simulink library "StdAnimationLibrary_R2020b"  (R2020b)
settings: Solver=VariableStepAuto  StartTime=0.0  StopTime=10.0  RelTol=1e-3
libraries: simulink x8
settings Model: Creator=mchawa  LastModifiedBy=oashraf
settings DataIOCC: ReturnWorkspaceOutputs=off
settings DebuggingCC: ArithmeticOperatorsInVariantConditions=warning
settings SFSimCC: SimUseLocalCustomCode=off  CustomCodeUndefinedFunction=UseInterfaceOnly
settings RTWCC: RTWUseLocalCustomCode=off

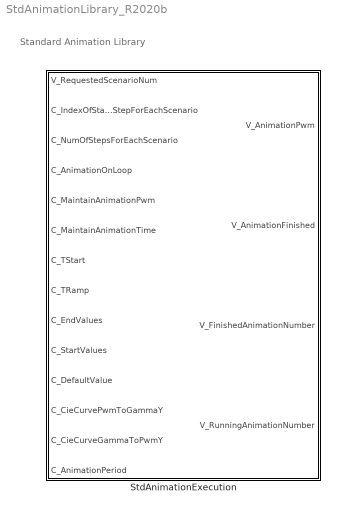
== system StdAnimationLibrary_R2020b ==
  note: Standard Animation Library
  StdAnimationExecution : Subsystem  Description=|
      | S___122_135
      | S___122_242
      | S___122_240

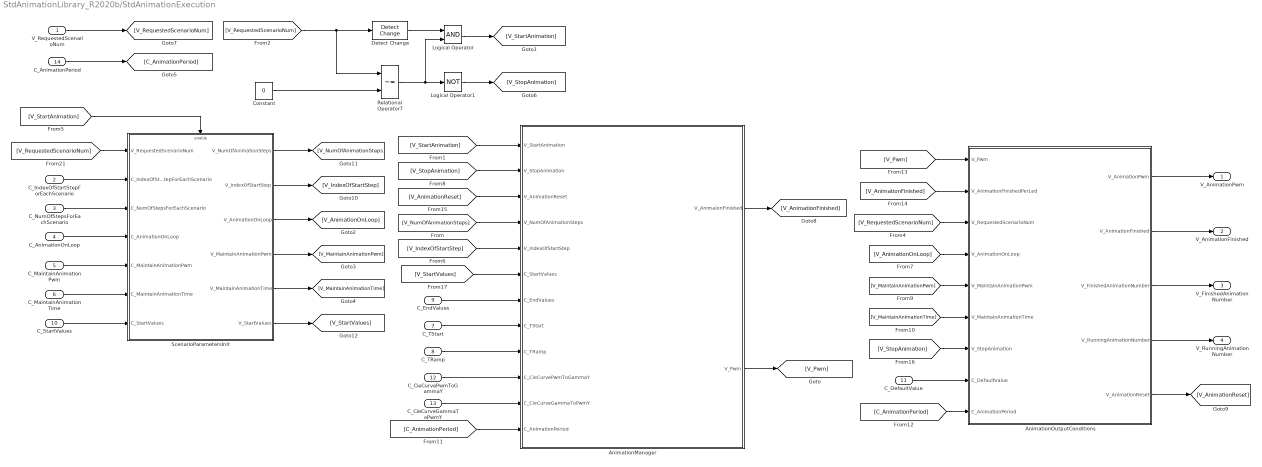
== system StdAnimationLibrary_R2020b/StdAnimationExecution ==
  V_RequestedScenarioNum : Inport
  C_IndexOfStartStepForEachScenario : Inport  Port=2
  C_NumOfStepsForEachScenario : Inport  Port=3
  C_AnimationOnLoop : Inport  Port=4
  C_MaintainAnimationPwm : Inport  Port=5
  C_MaintainAnimationTime : Inport  Port=6
  C_TStart : Inport  Port=7
  C_TRamp : Inport  Port=8
  C_EndValues : Inport  Port=9
  C_StartValues : Inport  Port=10
  C_DefaultValue : Inport  Port=11
  C_CieCurvePwmToGammaY : Inport  Port=12
  C_CieCurveGammaToPwmY : Inport  Port=13
  C_AnimationPeriod : Inport  Port=14
  AnimationManager : Subsystem  TreatAsAtomicUnit=on
  AnimationOutputConditions : Subsystem  Description=|
      | S___122_237
      | S___122_244
  Constant : Constant  Value=0  OutDataTypeStr=uint8
  Detect Change : simulink/Logic and Bit Operations/Detect Change  vinit=0  OutDataTypeStr=boolean
  Logical Operator : Logic  AllPortsSameDT=off  OutDataTypeStr=boolean
  Logical Operator1 : Logic  Operator=NOT  AllPortsSameDT=off  OutDataTypeStr=boolean
  Relational Operator7 : RelationalOperator  Operator=~=  OutDataTypeStr=boolean  RndMeth=Simplest
  ScenarioParametersInit : Subsystem  TreatAsAtomicUnit=on
  V_AnimationPwm : Outport  VectorParamsAs1DForOutWhenUnconnected=off
  V_AnimationFinished : Outport  Port=2  VectorParamsAs1DForOutWhenUnconnected=off
  V_FinishedAnimationNumber : Outport  Port=3  VectorParamsAs1DForOutWhenUnconnected=off
  V_RunningAnimationNumber : Outport  Port=4  VectorParamsAs1DForOutWhenUnconnected=off
  wires:
  V_RequestedScenarioNum/1 -> [V_RequestedScenarioNum]
  [V_StartAnimation] -> AnimationManager/1(V_StartAnimation)
  C_EndValues/1 -> AnimationManager/7(C_EndValues)
  C_TStart/1 -> AnimationManager/8(C_TStart)
  [V_StopAnimation] -> AnimationManager/2(V_StopAnimation)
  C_TRamp/1 -> AnimationManager/9(C_TRamp)
  Constant/1 -> Relational Operator7/2
  C_CieCurveGammaToPwmY/1 -> AnimationManager/11(C_CieCurveGammaToPwmY)
  [V_RequestedScenarioNum] -> AnimationOutputConditions/3(V_RequestedScenarioNum)
  [V_RequestedScenarioNum] -> Relational Operator7/1, Detect Change/1
  C_IndexOfStartStepForEachScenario/1 -> ScenarioParametersInit/2(C_IndexOfStartStepForEachScenario)
  C_NumOfStepsForEachScenario/1 -> ScenarioParametersInit/3(C_NumOfStepsForEachScenario)
  C_DefaultValue/1 -> AnimationOutputConditions/8(C_DefaultValue)
  C_CieCurvePwmToGammaY/1 -> AnimationManager/10(C_CieCurvePwmToGammaY)
  [V_RequestedScenarioNum] -> ScenarioParametersInit/1(V_RequestedScenarioNum)
  ScenarioParametersInit/2(V_IndexOfStartStep) -> [V_IndexOfStartStep]
  ScenarioParametersInit/1(V_NumOfAnimationSteps) -> [V_NumOfAnimationSteps]
  [V_StartAnimation] -> ScenarioParametersInit/Enable
  [V_NumOfAnimationSteps] -> AnimationManager/4(V_NumOfAnimationSteps)
  [V_IndexOfStartStep] -> AnimationManager/5(V_IndexOfStartStep)
  C_AnimationOnLoop/1 -> ScenarioParametersInit/4(C_AnimationOnLoop)
  C_MaintainAnimationPwm/1 -> ScenarioParametersInit/5(C_MaintainAnimationPwm)
  C_MaintainAnimationTime/1 -> ScenarioParametersInit/6(C_MaintainAnimationTime)
  Detect Change/1 -> Logical Operator/1
  Relational Operator7/1 -> Logical Operator1/1, Logical Operator/2
  Logical Operator/1 -> [V_StartAnimation]
  Logical Operator1/1 -> [V_StopAnimation]
  ScenarioParametersInit/3(V_AnimationOnLoop) -> [V_AnimationOnLoop]
  ScenarioParametersInit/4(V_MaintainAnimationPwm) -> [V_MaintainAnimationPwm]
  ScenarioParametersInit/5(V_MaintainAnimationTime) -> [V_MaintainAnimationTime]
  [V_AnimationOnLoop] -> AnimationOutputConditions/4(V_AnimationOnLoop)
  [V_MaintainAnimationPwm] -> AnimationOutputConditions/5(V_MaintainAnimationPwm)
  [V_MaintainAnimationTime] -> AnimationOutputConditions/6(V_MaintainAnimationTime)
  C_AnimationPeriod/1 -> [C_AnimationPeriod]
  [C_AnimationPeriod] -> AnimationManager/12(C_AnimationPeriod)
  [C_AnimationPeriod] -> AnimationOutputConditions/9(C_AnimationPeriod)
  AnimationManager/2(V_Pwm) -> [V_Pwm]
  AnimationManager/1(V_AnimaionFinished) -> [V_AnimationFinished]
  [V_Pwm] -> AnimationOutputConditions/1(V_Pwm)
  [V_AnimationFinished] -> AnimationOutputConditions/2(V_AnimationFinishedPerLed)
  [V_AnimationReset] -> AnimationManager/3(V_AnimationReset)
  [V_StopAnimation] -> AnimationOutputConditions/7(V_StopAnimation)
  C_StartValues/1 -> ScenarioParametersInit/7(C_StartValues)
  ScenarioParametersInit/6(V_StartValues) -> [V_StartValues]
  [V_StartValues] -> AnimationManager/6(C_StartValues)
  AnimationOutputConditions/1(V_AnimationPwm) -> V_AnimationPwm/1
  AnimationOutputConditions/3(V_FinishedAnimationNumber) -> V_FinishedAnimationNumber/1
  AnimationOutputConditions/4(V_RunningAnimationNumber) -> V_RunningAnimationNumber/1
  AnimationOutputConditions/5(V_AnimationReset) -> [V_AnimationReset]
  AnimationOutputConditions/2(V_AnimationFinished) -> V_AnimationFinished/1

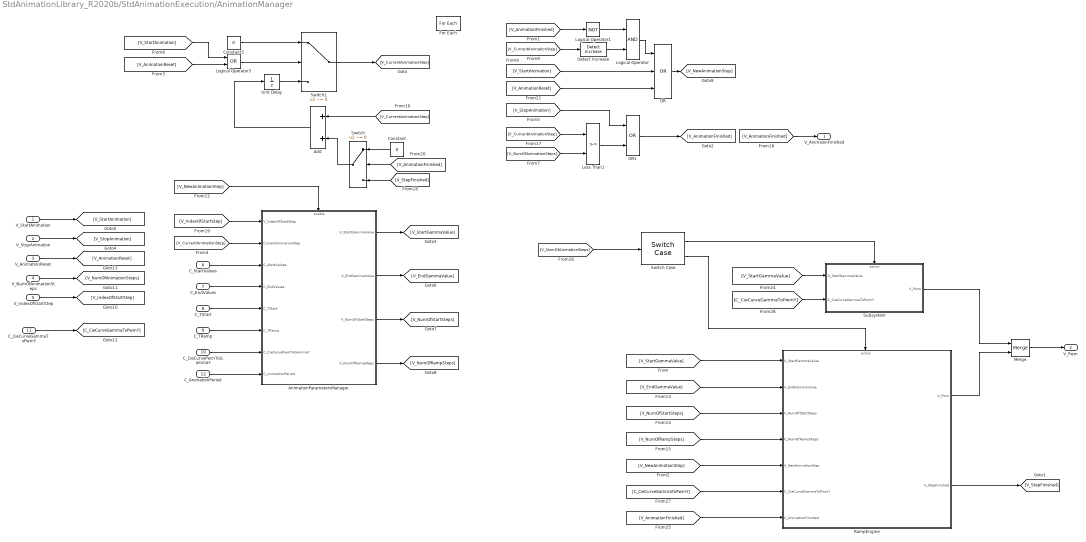
== system StdAnimationLibrary_R2020b/StdAnimationExecution/AnimationManager ==
  V_StartAnimation : Inport  OutDataTypeStr=boolean
  V_StopAnimation : Inport  Port=2  OutDataTypeStr=boolean
  V_AnimationReset : Inport  Port=3
  V_NumOfAnimationSteps : Inport  Port=4  Partition=on  PartitionDimension=2  PartitionWidth=1  PartitionOffset=0
  V_IndexOfStartStep : Inport  Port=5  Partition=on  PartitionDimension=2  PartitionWidth=1  PartitionOffset=0
  C_StartValues : Inport  Port=6  Partition=on  PartitionDimension=2  PartitionWidth=1  PartitionOffset=0
  C_EndValues : Inport  Port=7
  C_TStart : Inport  Port=8
  C_TRamp : Inport  Port=9
  C_CieCurvePwmToGammaY : Inport  Port=10
  C_CieCurveGammaToPwmY : Inport  Port=11
  C_AnimationPeriod : Inport  Port=12
  Add : Sum
  AnimationParametersManager : Subsystem  TreatAsAtomicUnit=on
  Constant : Constant  Value=0  OutDataTypeStr=uint8
  Constant5 : Constant  Value=0  OutDataTypeStr=uint8
  Detect Increase : simulink/Logic and Bit Operations/Detect Increase  vinit=0.0  OutDataTypeStr=boolean
  For Each : ForEach  DisableCoverage=on
  Less Than1 : RelationalOperator  OutDataTypeStr=boolean  RndMeth=Simplest
  Logical Operator : Logic  AllPortsSameDT=off  OutDataTypeStr=boolean
  Logical Operator1 : Logic  Operator=NOT  AllPortsSameDT=off  OutDataTypeStr=boolean
  Logical Operator3 : Logic  Operator=OR  AllPortsSameDT=off  OutDataTypeStr=boolean
  Merge : Merge
  OR : Logic  Operator=OR  Inputs=3  AllPortsSameDT=off  OutDataTypeStr=boolean
  OR1 : Logic  Operator=OR  AllPortsSameDT=off  OutDataTypeStr=boolean
  RampEngine : Subsystem
  Subsystem : Subsystem
  Switch : Switch  Criteria=u2 ~= 0
  Switch Case : SwitchCase  CaseConditions={0}
  Switch1 : Switch  Criteria=u2 ~= 0  OutDataTypeStr=Inherit: Inherit via back propagation  SaturateOnIntegerOverflow=on
  Unit Delay : UnitDelay  SampleTime=-1  HasFrameUpgradeWarning=on
  V_AnimaionFinished : Outport  ConcatenationDimension=1  VectorParamsAs1DForOutWhenUnconnected=off
  V_Pwm : Outport  Port=2  ConcatenationDimension=1  VectorParamsAs1DForOutWhenUnconnected=off
  wires:
  [V_CurrentAnimationStep] -> AnimationParametersManager/2(CurrentAnimationStep)
  Constant5/1 -> Switch1/1
  C_EndValues/1 -> AnimationParametersManager/4(C_EndValues)
  [V_StopAnimation] -> OR1/1
  C_TStart/1 -> AnimationParametersManager/5(C_TStart)
  C_TRamp/1 -> AnimationParametersManager/6(C_TRamp)
  V_StartAnimation/1 -> [V_StartAnimation]
  V_StopAnimation/1 -> [V_StopAnimation]
  C_StartValues/1 -> AnimationParametersManager/3(C_StartValues)
  Switch1/1 -> [V_CurrentAnimationStep]
  RampEngine/1(V_Pwm) -> Merge/2
  Add/1 -> Unit Delay/1
  [V_StartAnimation] -> OR/2
  [V_NewAnimationStep] -> AnimationParametersManager/Enable
  C_AnimationPeriod/1 -> AnimationParametersManager/8(C_AnimationPeriod)
  AnimationParametersManager/1(V_StartGammaValue) -> [V_StartGammaValue]
  AnimationParametersManager/2(V_EndGammaValue) -> [V_EndGammaValue]
  AnimationParametersManager/3(V_NumOfStartSteps) -> [V_NumOfStartSteps]
  AnimationParametersManager/4(V_NumOfRampSteps) -> [V_NumOfRampSteps]
  [V_NewAnimationStep] -> RampEngine/5(V_NewAnimationStep)
  [V_StartGammaValue] -> RampEngine/1(V_StartGammaValue)
  [V_EndGammaValue] -> RampEngine/2(V_EndGammaValue)
  [V_NumOfStartSteps] -> RampEngine/3(V_NumOfStartSteps)
  [V_NumOfRampSteps] -> RampEngine/4(V_NumOfRampSteps)
  [V_AnimationFinished] -> V_AnimaionFinished/1
  [V_CurrentAnimationStep] -> Detect Increase/1
  Logical Operator/1 -> OR/1
  Logical Operator1/1 -> Logical Operator/1
  [V_AnimationFinished] -> Logical Operator1/1
  RampEngine/2(V_StepFinished) -> [V_StepFinished]
  [V_CurrentAnimationStep] -> Add/1
  Unit Delay/1 -> Switch1/3
  Less Than1/1 -> OR1/2
  OR/1 -> [V_NewAnimationStep]
  OR1/1 -> [V_AnimationFinished]
  Detect Increase/1 -> Logical Operator/2
  [V_IndexOfStartStep] -> AnimationParametersManager/1(V_IndexOfStartStep)
  Switch/1 -> Add/2
  [V_StepFinished] -> Switch/3
  [V_AnimationFinished] -> Switch/2
  Constant/1 -> Switch/1
  [V_NumOfAnimationSteps] -> Less Than1/2
  [V_CurrentAnimationStep] -> Less Than1/1
  C_CieCurvePwmToGammaY/1 -> AnimationParametersManager/7(C_CieCurvePwmToGammaY)
  V_IndexOfStartStep/1 -> [V_IndexOfStartStep]
  V_NumOfAnimationSteps/1 -> [V_NumOfAnimationSteps]
  V_AnimationReset/1 -> [V_AnimationReset]
  Logical Operator3/1 -> Switch1/2
  [V_AnimationReset] -> Logical Operator3/2
  [V_StartAnimation] -> Logical Operator3/1
  [V_AnimationReset] -> OR/3
  Subsystem/1(V_Pwm) -> Merge/1
  [V_StartGammaValue] -> Subsystem/1(V_StartGammaValue)
  [V_NumOfAnimationSteps] -> Switch Case/1
  Switch Case/1 -> Subsystem/Action
  [V_AnimationFinished] -> RampEngine/7(V_AnimationFinished)
  Merge/1 -> V_Pwm/1
  C_CieCurveGammaToPwmY/1 -> [C_CieCurveGammaToPwmY]
  [C_CieCurveGammaToPwmY] -> RampEngine/6(C_CieCurveGammaToPwmY)
  [C_CieCurveGammaToPwmY] -> Subsystem/2(C_CieCurveGammaToPwmY)
  Switch Case/2 -> RampEngine/Action

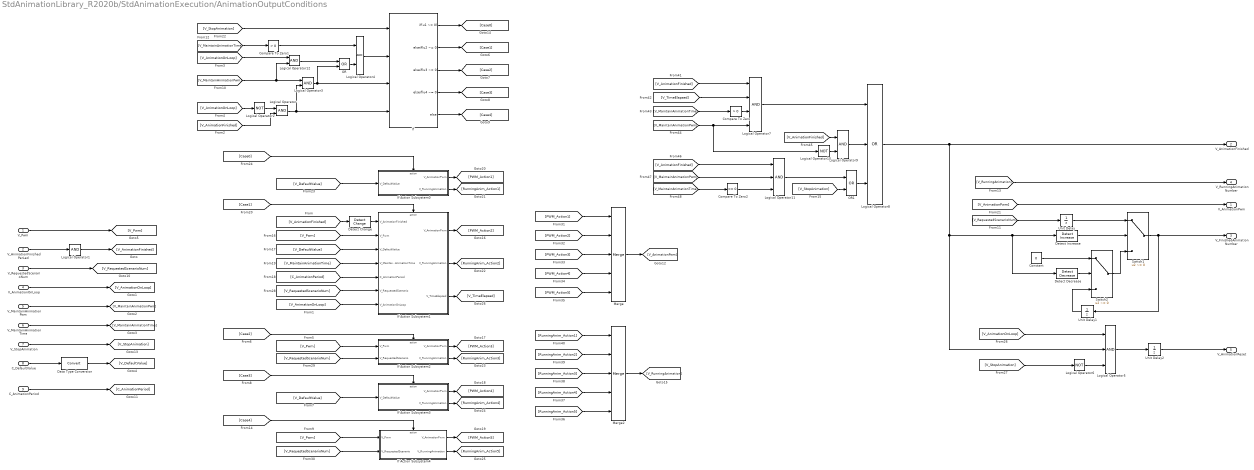
== system StdAnimationLibrary_R2020b/StdAnimationExecution/AnimationOutputConditions ==
  V_Pwm : Inport
  V_AnimationFinishedPerLed : Inport  Port=2
  V_RequestedScenarioNum : Inport  Port=3
  V_AnimationOnLoop : Inport  Port=4
  V_MaintainAnimationPwm : Inport  Port=5
  V_MaintainAnimationTime : Inport  Port=6
  V_StopAnimation : Inport  Port=7
  C_DefaultValue : Inport  Port=8
  C_AnimationPeriod : Inport  Port=9
  Compare To Zero : simulink/Logic and Bit Operations/Compare To Zero  relop=>  OutDataTypeStr=boolean
  Compare To Zero1 : simulink/Logic and Bit Operations/Compare To Zero  relop=>  OutDataTypeStr=boolean
  Compare To Zero2 : simulink/Logic and Bit Operations/Compare To Zero  relop===  OutDataTypeStr=boolean
  Constant : Constant  Value=0  OutDataTypeStr=uint8
  Data Type Conversion : DataTypeConversion
  Detect Change : simulink/Logic and Bit Operations/Detect Change  vinit=0  OutDataTypeStr=boolean
  Detect Decrease : simulink/Logic and Bit Operations/Detect Decrease  vinit=0.0  OutDataTypeStr=boolean
  Detect Increase : simulink/Logic and Bit Operations/Detect Increase  vinit=0.0  OutDataTypeStr=boolean
  If : If  NumInputs=4  IfExpression=u1 ~= 0  ElseIfExpressions=u2 ~= 0, u3 ~= 0, u4 ~= 0
  If Action Subsystem0 : Subsystem  TreatAsAtomicUnit=on
  If Action Subsystem1 : Subsystem  Description=S___122_238  TreatAsAtomicUnit=on
  If Action Subsystem2 : Subsystem  TreatAsAtomicUnit=on
  If Action Subsystem3 : Subsystem  TreatAsAtomicUnit=on
  If Action Subsystem4 : Subsystem  TreatAsAtomicUnit=on
  Logical Operator{,3..4,9,12} (5 alike) : Logic  AllPortsSameDT=off  OutDataTypeStr=boolean
  Logical Operator1 : Logic  Inputs=1  AllPortsSameDT=off  OutDataTypeStr=boolean
  Logical Operator10 : Logic  Operator=NOT  AllPortsSameDT=off  OutDataTypeStr=boolean
  Logical Operator11 : Logic  Inputs=3  AllPortsSameDT=off  OutDataTypeStr=boolean
  Logical Operator2 : Logic  Operator=NOT  AllPortsSameDT=off  OutDataTypeStr=boolean
  Logical Operator5 : Logic  Inputs=3  AllPortsSameDT=off  OutDataTypeStr=boolean
  Logical Operator6 : Logic  Operator=NOT  AllPortsSameDT=off  OutDataTypeStr=boolean
  Logical Operator7 : Logic  Inputs=4  AllPortsSameDT=off  OutDataTypeStr=boolean
  Logical Operator8 : Logic  Operator=OR  Inputs=3  AllPortsSameDT=off  OutDataTypeStr=boolean
  Merge : Merge  Inputs=5
  Merge2 : Merge  Inputs=5
  OR : Logic  Operator=OR  AllPortsSameDT=off  OutDataTypeStr=boolean
  OR1 : Logic  Operator=OR  AllPortsSameDT=off  OutDataTypeStr=boolean
  Switch1 : Switch  Criteria=u2 ~= 0
  Switch2 : Switch  Criteria=u2 ~= 0
  Unit Delay : UnitDelay  SampleTime=-1  HasFrameUpgradeWarning=on
  Unit Delay1 : UnitDelay  SampleTime=-1  HasFrameUpgradeWarning=on
  Unit Delay2 : UnitDelay  SampleTime=-1  HasFrameUpgradeWarning=on
  V_AnimationPwm : Outport
  V_AnimationFinished : Outport  Port=2
  V_FinishedAnimationNumber : Outport  Port=3
  V_RunningAnimationNumber : Outport  Port=4
  V_AnimationReset : Outport  Port=5
  wires:
  [V_StopAnimation] -> OR1/2
  Logical Operator11/1 -> OR1/1
  OR1/1 -> Logical Operator8/3
  V_AnimationFinishedPerLed/1 -> Logical Operator1/1
  V_RequestedScenarioNum/1 -> [V_RequestedScenarioNum]
  [V_RequestedScenarioNum] -> Unit Delay/1
  C_DefaultValue/1 -> Data Type Conversion/1
  Logical Operator1/1 -> [V_AnimationFinished]
  Unit Delay/1 -> Switch1/1
  Switch2/1 -> Switch1/3
  Switch1/1 -> V_FinishedAnimationNumber/1, Unit Delay1/1
  Unit Delay1/1 -> Switch2/3
  Detect Increase/1 -> Switch1/2
  Detect Decrease/1 -> Switch2/2
  Constant/1 -> Switch2/1
  [V_AnimationFinished] -> Logical Operator/2
  [V_AnimationOnLoop] -> Logical Operator2/1
  V_AnimationOnLoop/1 -> [V_AnimationOnLoop]
  V_MaintainAnimationPwm/1 -> [V_MaintainAnimationPwm]
  V_MaintainAnimationTime/1 -> [V_MaintainAnimationTime]
  Data Type Conversion/1 -> [V_DefaultValue]
  V_Pwm/1 -> [V_Pwm]
  Logical Operator2/1 -> Logical Operator/1
  [V_MaintainAnimationPwm] -> Logical Operator12/2, Logical Operator3/1
  Logical Operator3/1 -> OR/2, If/3
  [V_MaintainAnimationTime] -> Compare To Zero1/1
  Compare To Zero1/1 -> Logical Operator4/1
  If/5 -> [Case4]
  [V_Pwm] -> If Action Subsystem2/1(V_Pwm)
  [Case2] -> If Action Subsystem2/Action
  [V_DefaultValue] -> If Action Subsystem3/1(V_DefaultValue)
  [Case3] -> If Action Subsystem3/Action
  [V_Pwm] -> If Action Subsystem4/1(V_Pwm)
  [Case4] -> If Action Subsystem4/Action
  C_AnimationPeriod/1 -> [C_AnimationPeriod]
  [V_Pwm] -> If Action Subsystem1/2(V_Pwm)
  [V_DefaultValue] -> If Action Subsystem1/3(V_DefaultValue)
  [V_MaintainAnimationTime] -> If Action Subsystem1/4(V_MaintainAnimationTime)
  [C_AnimationPeriod] -> If Action Subsystem1/5(C_AnimationPeriod)
  [Case1] -> If Action Subsystem1/Action
  Merge/1 -> [V_AnimationPwm]
  [V_AnimationPwm] -> V_AnimationPwm/1
  V_StopAnimation/1 -> [V_StopAnimation]
  If/4 -> [Case3]
  If/1 -> [Case0]
  If/2 -> [Case1]
  If/3 -> [Case2]
  [V_StopAnimation] -> If/1
  Logical Operator4/1 -> If/2
  Logical Operator/1 -> Logical Operator3/2, If/4
  [V_DefaultValue] -> If Action Subsystem0/1(V_DefaultValue)
  [Case0] -> If Action Subsystem0/Action
  [V_AnimationOnLoop] -> Logical Operator5/1
  [V_StopAnimation] -> Logical Operator6/1
  Logical Operator6/1 -> Logical Operator5/3
  Logical Operator5/1 -> Unit Delay2/1
  Unit Delay2/1 -> V_AnimationReset/1
  [V_RunningAnimation] -> V_RunningAnimationNumber/1
  [V_RequestedScenarioNum] -> If Action Subsystem1/6(V_RequestedScenario)
  [V_RequestedScenarioNum] -> If Action Subsystem2/2(V_RequestedScenario)
  [V_RequestedScenarioNum] -> If Action Subsystem4/2(V_RequestedScenario)
  Merge2/1 -> [V_RunningAnimation]
  If Action Subsystem2/1(V_AnimationPwm) -> [PWM_Action3]
  If Action Subsystem1/1(V_AnimationPwm) -> [PWM_Action2]
  If Action Subsystem3/1(V_AnimationPwm) -> [PWM_Action4]
  If Action Subsystem4/1(V_AnimationPwm) -> [PWM_Action5]
  If Action Subsystem0/1(V_AnimationPwm) -> [PWM_Action1]
  [PWM_Action1] -> Merge/1
  [PWM_Action2] -> Merge/2
  [PWM_Action3] -> Merge/3
  [PWM_Action4] -> Merge/4
  [PWM_Action5] -> Merge/5
  If Action Subsystem0/2(V_RunningAnimation) -> [RunningAnim_Action1]
  If Action Subsystem1/2(V_RunningAnimation) -> [RunningAnim_Action2]
  If Action Subsystem2/2(V_RunningAnimation) -> [RunningAnim_Action3]
  If Action Subsystem3/2(V_RunningAnimation) -> [RunningAnim_Action4]
  If Action Subsystem4/2(V_RunningAnimation) -> [RunningAnim_Action5]
  [RunningAnim_Action1] -> Merge2/1
  [RunningAnim_Action2] -> Merge2/2
  [RunningAnim_Action3] -> Merge2/3
  [RunningAnim_Action4] -> Merge2/4
  [RunningAnim_Action5] -> Merge2/5
  [V_TimeElapsed] -> Logical Operator7/2
  [V_MaintainAnimationTime] -> Compare To Zero/1
  Compare To Zero2/1 -> Logical Operator11/3
  Logical Operator7/1 -> Logical Operator8/1
  [V_AnimationFinished] -> Logical Operator11/1
  [V_MaintainAnimationPwm] -> Logical Operator7/4, Logical Operator10/1
  Logical Operator10/1 -> Logical Operator9/2
  Compare To Zero/1 -> Logical Operator7/3
  [V_MaintainAnimationTime] -> Compare To Zero2/1
  [V_MaintainAnimationPwm] -> Logical Operator11/2
  [V_AnimationFinished] -> Logical Operator9/1
  Logical Operator9/1 -> Logical Operator8/2
  [V_AnimationFinished] -> Logical Operator7/1
  [V_AnimationFinished] -> Detect Change/1
  If Action Subsystem1/3(V_TimeElapsed) -> [V_TimeElapsed]
  Logical Operator8/1 -> Logical Operator5/2, Detect Increase/1, Detect Decrease/1, V_AnimationFinished/1
  OR/1 -> Logical Operator4/2
  [V_AnimationOnLoop] -> If Action Subsystem1/7(V_AnimationOnLoop)
  Detect Change/1 -> If Action Subsystem1/1(V_AnimationFinished)
  [V_AnimationOnLoop] -> Logical Operator12/1
  Logical Operator12/1 -> OR/1

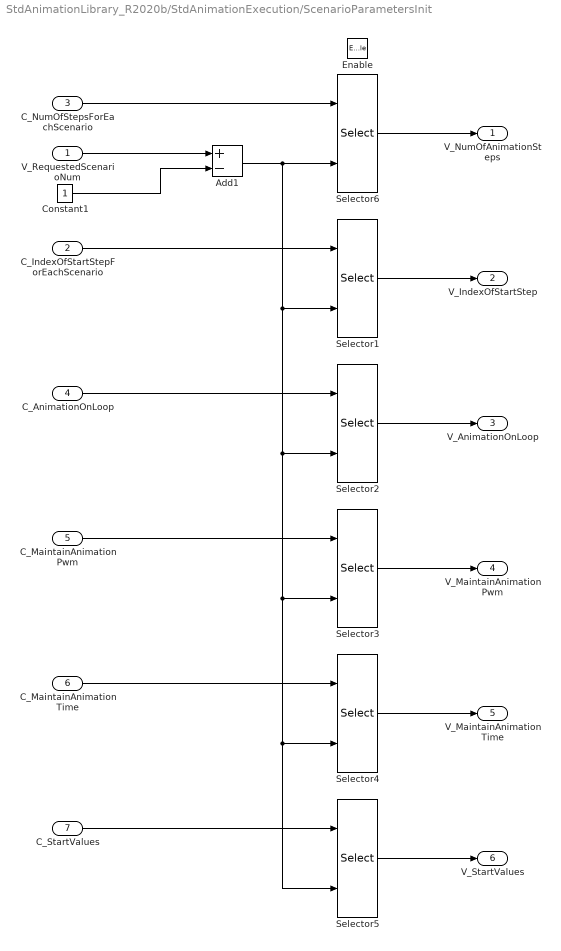
== system StdAnimationLibrary_R2020b/StdAnimationExecution/ScenarioParametersInit ==
  V_RequestedScenarioNum : Inport
  C_IndexOfStartStepForEachScenario : Inport  Port=2
  C_NumOfStepsForEachScenario : Inport  Port=3
  C_AnimationOnLoop : Inport  Port=4
  C_MaintainAnimationPwm : Inport  Port=5
  C_MaintainAnimationTime : Inport  Port=6
  C_StartValues : Inport  Port=7
  Enable : EnablePort
  Add1 : Sum  Inputs=+-  OutDataTypeStr=Inherit: Inherit via back propagation  SaturateOnIntegerOverflow=on
  Constant1 : Constant  OutDataTypeStr=uint8
  Selector1 : Selector  NumberOfDimensions=2  IndexMode=Zero-based  IndexOptions=Index vector (port),Select all  Indices=[1 3],1  OutputSizes=1,1
  Selector2 : Selector  IndexMode=Zero-based  IndexOptions=Index vector (port)  Indices=[1 3]  OutputSizes=1
  Selector3 : Selector  IndexMode=Zero-based  IndexOptions=Index vector (port)  Indices=[1 3]  OutputSizes=1
  Selector4 : Selector  IndexMode=Zero-based  IndexOptions=Index vector (port)  Indices=[1 3]  OutputSizes=1
  Selector5 : Selector  NumberOfDimensions=2  IndexMode=Zero-based  IndexOptions=Index vector (port),Select all  Indices=[1 3],1  OutputSizes=1,1
  Selector6 : Selector  NumberOfDimensions=2  IndexMode=Zero-based  IndexOptions=Index vector (port),Select all  Indices=[1 3],1  OutputSizes=1,1
  V_NumOfAnimationSteps : Outport  InitialOutput=0  VectorParamsAs1DForOutWhenUnconnected=off
  V_IndexOfStartStep : Outport  Port=2  InitialOutput=0  VectorParamsAs1DForOutWhenUnconnected=off
  V_AnimationOnLoop : Outport  Port=3  InitialOutput=0  VectorParamsAs1DForOutWhenUnconnected=off
  V_MaintainAnimationPwm : Outport  Port=4  InitialOutput=0  VectorParamsAs1DForOutWhenUnconnected=off
  V_MaintainAnimationTime : Outport  Port=5  InitialOutput=0  VectorParamsAs1DForOutWhenUnconnected=off
  V_StartValues : Outport  Port=6  InitialOutput=0  VectorParamsAs1DForOutWhenUnconnected=off
  wires:
  C_NumOfStepsForEachScenario/1 -> Selector6/1
  Selector6/1 -> V_NumOfAnimationSteps/1
  C_IndexOfStartStepForEachScenario/1 -> Selector1/1
  Selector1/1 -> V_IndexOfStartStep/1
  Constant1/1 -> Add1/2
  Add1/1 -> Selector5/2, Selector4/2, Selector3/2, Selector2/2, Selector1/2, Selector6/2
  V_RequestedScenarioNum/1 -> Add1/1
  C_AnimationOnLoop/1 -> Selector2/1
  Selector2/1 -> V_AnimationOnLoop/1
  C_MaintainAnimationPwm/1 -> Selector3/1
  C_MaintainAnimationTime/1 -> Selector4/1
  Selector3/1 -> V_MaintainAnimationPwm/1
  Selector4/1 -> V_MaintainAnimationTime/1
  C_StartValues/1 -> Selector5/1
  Selector5/1 -> V_StartValues/1

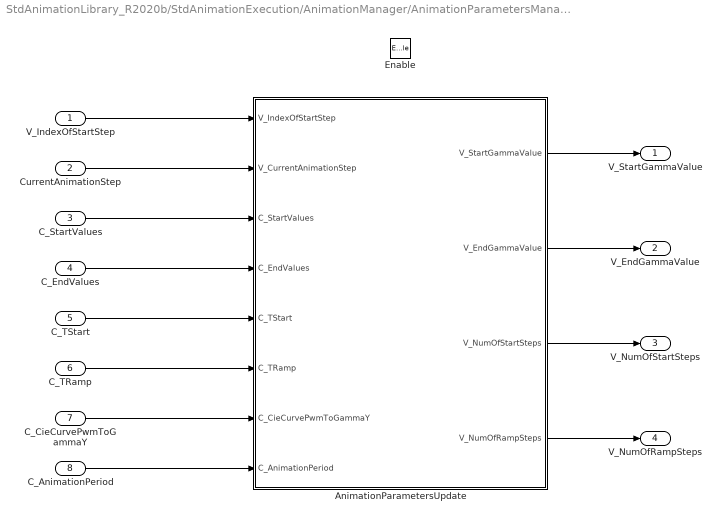
== system StdAnimationLibrary_R2020b/StdAnimationExecution/AnimationManager/AnimationParametersManager ==
  V_IndexOfStartStep : Inport
  CurrentAnimationStep : Inport  Port=2
  C_StartValues : Inport  Port=3
  C_EndValues : Inport  Port=4
  C_TStart : Inport  Port=5
  C_TRamp : Inport  Port=6
  C_CieCurvePwmToGammaY : Inport  Port=7
  C_AnimationPeriod : Inport  Port=8
  Enable : EnablePort
  AnimationParametersUpdate : Subsystem  TreatAsAtomicUnit=on
  V_StartGammaValue : Outport  InitialOutput=0  VectorParamsAs1DForOutWhenUnconnected=off
  V_EndGammaValue : Outport  Port=2  InitialOutput=0  VectorParamsAs1DForOutWhenUnconnected=off
  V_NumOfStartSteps : Outport  Port=3  InitialOutput=0  VectorParamsAs1DForOutWhenUnconnected=off
  V_NumOfRampSteps : Outport  Port=4  InitialOutput=0  VectorParamsAs1DForOutWhenUnconnected=off
  wires:
  C_EndValues/1 -> AnimationParametersUpdate/4(C_EndValues)
  C_TStart/1 -> AnimationParametersUpdate/5(C_TStart)
  C_TRamp/1 -> AnimationParametersUpdate/6(C_TRamp)
  AnimationParametersUpdate/1(V_StartGammaValue) -> V_StartGammaValue/1
  AnimationParametersUpdate/2(V_EndGammaValue) -> V_EndGammaValue/1
  AnimationParametersUpdate/3(V_NumOfStartSteps) -> V_NumOfStartSteps/1
  AnimationParametersUpdate/4(V_NumOfRampSteps) -> V_NumOfRampSteps/1
  C_StartValues/1 -> AnimationParametersUpdate/3(C_StartValues)
  CurrentAnimationStep/1 -> AnimationParametersUpdate/2(V_CurrentAnimationStep)
  V_IndexOfStartStep/1 -> AnimationParametersUpdate/1(V_IndexOfStartStep)
  C_AnimationPeriod/1 -> AnimationParametersUpdate/8(C_AnimationPeriod)
  C_CieCurvePwmToGammaY/1 -> AnimationParametersUpdate/7(C_CieCurvePwmToGammaY)

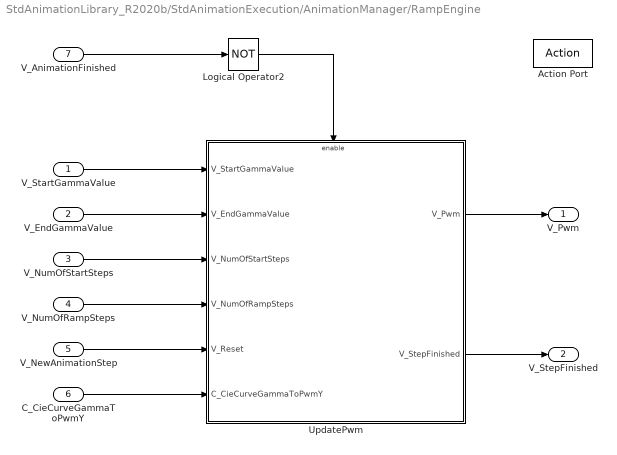
== system StdAnimationLibrary_R2020b/StdAnimationExecution/AnimationManager/RampEngine ==
  V_StartGammaValue : Inport
  V_EndGammaValue : Inport  Port=2
  V_NumOfStartSteps : Inport  Port=3
  V_NumOfRampSteps : Inport  Port=4
  V_NewAnimationStep : Inport  Port=5  OutDataTypeStr=boolean
  C_CieCurveGammaToPwmY : Inport  Port=6
  V_AnimationFinished : Inport  Port=7
  Action Port : ActionPort
  Logical Operator2 : Logic  Operator=NOT  AllPortsSameDT=off  OutDataTypeStr=boolean
  UpdatePwm : Subsystem  TreatAsAtomicUnit=on
  V_Pwm : Outport  InitialOutput=0  VectorParamsAs1DForOutWhenUnconnected=off
  V_StepFinished : Outport  Port=2  InitialOutput=0  VectorParamsAs1DForOutWhenUnconnected=off
  wires:
  V_StartGammaValue/1 -> UpdatePwm/1(V_StartGammaValue)
  UpdatePwm/1(V_Pwm) -> V_Pwm/1
  UpdatePwm/2(V_StepFinished) -> V_StepFinished/1
  C_CieCurveGammaToPwmY/1 -> UpdatePwm/6(C_CieCurveGammaToPwmY)
  V_EndGammaValue/1 -> UpdatePwm/2(V_EndGammaValue)
  V_NumOfStartSteps/1 -> UpdatePwm/3(V_NumOfStartSteps)
  V_NumOfRampSteps/1 -> UpdatePwm/4(V_NumOfRampSteps)
  V_NewAnimationStep/1 -> UpdatePwm/5(V_Reset)
  V_AnimationFinished/1 -> Logical Operator2/1
  Logical Operator2/1 -> UpdatePwm/Enable

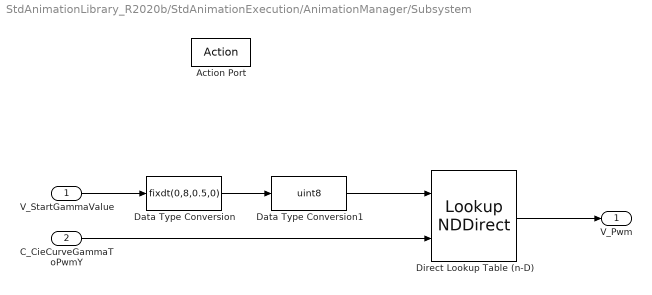
== system StdAnimationLibrary_R2020b/StdAnimationExecution/AnimationManager/Subsystem ==
  V_StartGammaValue : Inport
  C_CieCurveGammaToPwmY : Inport  Port=2
  Action Port : ActionPort
  Data Type Conversion : DataTypeConversion  OutDataTypeStr=fixdt(0,8,0.5,0)  RndMeth=Round
  Data Type Conversion1 : DataTypeConversion  OutDataTypeStr=uint8  ConvertRealWorld=Stored Integer (SI)
  Direct Lookup Table (n-D) : LookupNDDirect  NumberOfTableDimensions=1  TableIsInput=on  RemoveProtectionInput=on
  V_Pwm : Outport  InitialOutput=0  VectorParamsAs1DForOutWhenUnconnected=off
  wires:
  Direct Lookup Table (n-D)/1 -> V_Pwm/1
  Data Type Conversion/1 -> Data Type Conversion1/1
  V_StartGammaValue/1 -> Data Type Conversion/1
  Data Type Conversion1/1 -> Direct Lookup Table (n-D)/1
  C_CieCurveGammaToPwmY/1 -> Direct Lookup Table (n-D)/2

== system StdAnimationLibrary_R2020b/StdAnimationExecution/AnimationOutputConditions/If Action Subsystem0 ==
  V_DefaultValue : Inport
  Action Port : ActionPort
  Constant : Constant  Value=0  OutDataTypeStr=uint8
  V_AnimationPwm : Outport
  V_RunningAnimation : Outport  Port=2
  wires:
  V_DefaultValue/1 -> V_AnimationPwm/1
  Constant/1 -> V_RunningAnimation/1

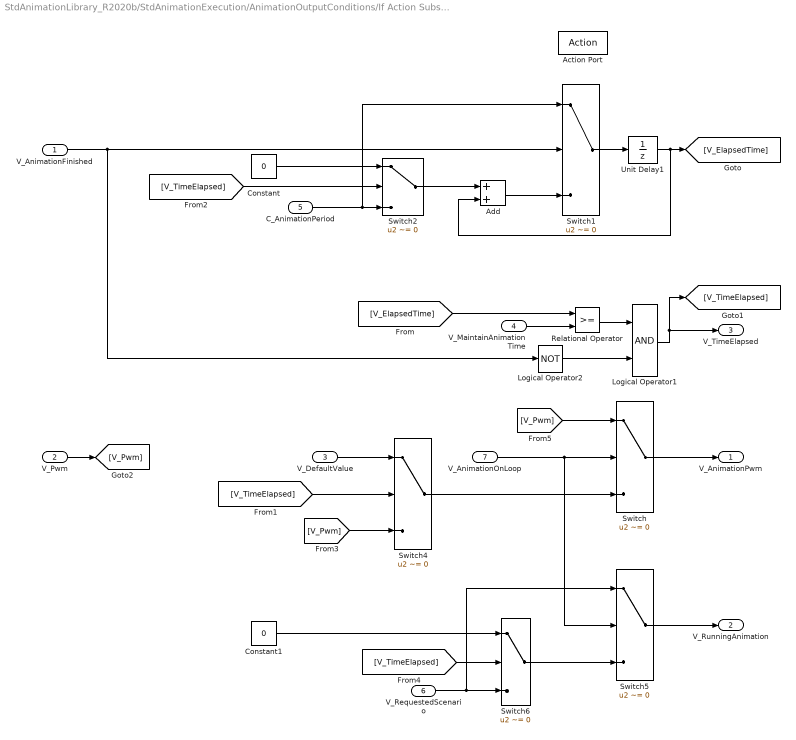
== system StdAnimationLibrary_R2020b/StdAnimationExecution/AnimationOutputConditions/If Action Subsystem1 ==
  V_AnimationFinished : Inport
  V_Pwm : Inport  Port=2
  V_DefaultValue : Inport  Port=3
  V_MaintainAnimationTime : Inport  Port=4
  C_AnimationPeriod : Inport  Port=5
  V_RequestedScenario : Inport  Port=6
  V_AnimationOnLoop : Inport  Port=7
  Action Port : ActionPort
  Add : Sum
  Constant : Constant  Value=0  OutDataTypeStr=Inherit: Inherit via back propagation
  Constant1 : Constant  Value=0  OutDataTypeStr=Inherit: Inherit via back propagation
  Logical Operator1 : Logic  AllPortsSameDT=off  OutDataTypeStr=boolean
  Logical Operator2 : Logic  Operator=NOT  AllPortsSameDT=off  OutDataTypeStr=boolean
  Relational Operator : RelationalOperator  OutDataTypeStr=boolean  RndMeth=Simplest
  Switch : Switch  Criteria=u2 ~= 0  OutDataTypeStr=Inherit: Inherit via back propagation  SaturateOnIntegerOverflow=on
  Switch1 : Switch  Criteria=u2 ~= 0
  Switch2 : Switch  Criteria=u2 ~= 0
  Switch4 : Switch  Criteria=u2 ~= 0  OutDataTypeStr=Inherit: Inherit via back propagation  SaturateOnIntegerOverflow=on
  Switch5 : Switch  Criteria=u2 ~= 0  OutDataTypeStr=Inherit: Inherit via back propagation  SaturateOnIntegerOverflow=on
  Switch6 : Switch  Criteria=u2 ~= 0
  Unit Delay1 : UnitDelay  SampleTime=-1  HasFrameUpgradeWarning=on
  V_AnimationPwm : Outport
  V_RunningAnimation : Outport  Port=2
  V_TimeElapsed : Outport  Port=3
  wires:
  Switch/1 -> V_AnimationPwm/1
  Constant/1 -> Switch2/1
  Switch1/1 -> Unit Delay1/1
  [V_ElapsedTime] -> Relational Operator/1
  V_MaintainAnimationTime/1 -> Relational Operator/2
  Add/1 -> Switch1/3
  Unit Delay1/1 -> [V_ElapsedTime], Add/2
  Switch2/1 -> Add/1
  [V_TimeElapsed] -> Switch2/2
  Constant1/1 -> Switch6/1
  Relational Operator/1 -> Logical Operator1/1
  Logical Operator1/1 -> V_TimeElapsed/1, [V_TimeElapsed]
  Logical Operator2/1 -> Logical Operator1/2
  V_AnimationFinished/1 -> Logical Operator2/1, Switch1/2
  V_AnimationOnLoop/1 -> Switch/2, Switch5/2
  Switch4/1 -> Switch/3
  V_DefaultValue/1 -> Switch4/1
  [V_TimeElapsed] -> Switch4/2
  [V_Pwm] -> Switch4/3
  Switch5/1 -> V_RunningAnimation/1
  Switch6/1 -> Switch5/3
  V_RequestedScenario/1 -> Switch6/3, Switch5/1
  [V_TimeElapsed] -> Switch6/2
  V_Pwm/1 -> [V_Pwm]
  [V_Pwm] -> Switch/1
  C_AnimationPeriod/1 -> Switch2/3, Switch1/1

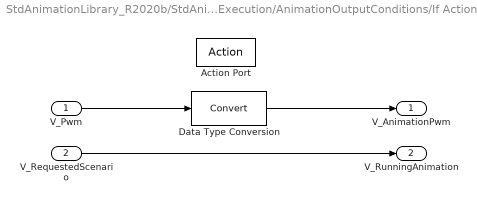
== system StdAnimationLibrary_R2020b/StdAnimationExecution/AnimationOutputConditions/If Action Subsystem2 ==
  V_Pwm : Inport
  V_RequestedScenario : Inport  Port=2
  Action Port : ActionPort
  Data Type Conversion : DataTypeConversion  SaturateOnIntegerOverflow=on
  V_AnimationPwm : Outport
  V_RunningAnimation : Outport  Port=2
  wires:
  V_Pwm/1 -> Data Type Conversion/1
  Data Type Conversion/1 -> V_AnimationPwm/1
  V_RequestedScenario/1 -> V_RunningAnimation/1

== system StdAnimationLibrary_R2020b/StdAnimationExecution/AnimationOutputConditions/If Action Subsystem3 ==
  V_DefaultValue : Inport
  Action Port : ActionPort
  Constant : Constant  Value=0  OutDataTypeStr=uint8
  V_AnimationPwm : Outport
  V_RunningAnimation : Outport  Port=2
  wires:
  V_DefaultValue/1 -> V_AnimationPwm/1
  Constant/1 -> V_RunningAnimation/1

== system StdAnimationLibrary_R2020b/StdAnimationExecution/AnimationOutputConditions/If Action Subsystem4 ==
  V_Pwm : Inport
  V_RequestedScenario : Inport  Port=2
  Action Port : ActionPort
  Data Type Conversion : DataTypeConversion  SaturateOnIntegerOverflow=on
  V_AnimationPwm : Outport
  V_RunningAnimation : Outport  Port=2
  wires:
  V_Pwm/1 -> Data Type Conversion/1
  Data Type Conversion/1 -> V_AnimationPwm/1
  V_RequestedScenario/1 -> V_RunningAnimation/1

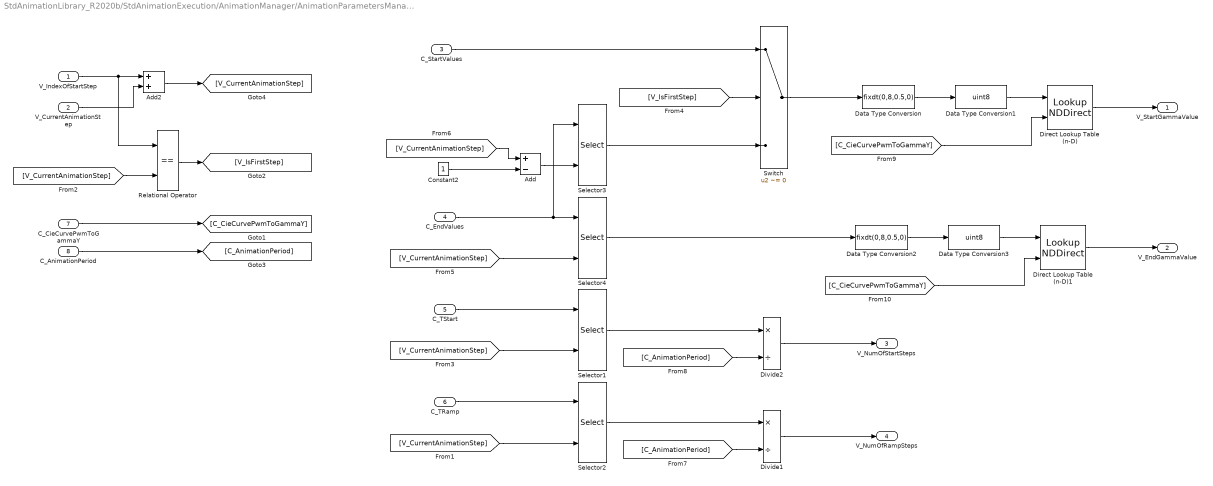
== system StdAnimationLibrary_R2020b/StdAnimationExecution/AnimationManager/AnimationParametersManager/AnimationParametersUpdate ==
  V_IndexOfStartStep : Inport
  V_CurrentAnimationStep : Inport  Port=2  OutDataTypeStr=uint8
  C_StartValues : Inport  Port=3
  C_EndValues : Inport  Port=4
  C_TStart : Inport  Port=5
  C_TRamp : Inport  Port=6
  C_CieCurvePwmToGammaY : Inport  Port=7
  C_AnimationPeriod : Inport  Port=8
  Add : Sum  Inputs=+-  OutDataTypeStr=Inherit: Inherit via back propagation  SaturateOnIntegerOverflow=on
  Add2 : Sum  OutDataTypeStr=Inherit: Inherit via back propagation  SaturateOnIntegerOverflow=on
  Constant2 : Constant  OutDataTypeStr=uint8
  Data Type Conversion : DataTypeConversion  OutDataTypeStr=fixdt(0,8,0.5,0)  RndMeth=Round
  Data Type Conversion1 : DataTypeConversion  OutDataTypeStr=uint8  ConvertRealWorld=Stored Integer (SI)
  Data Type Conversion2 : DataTypeConversion  OutDataTypeStr=fixdt(0,8,0.5,0)  RndMeth=Round
  Data Type Conversion3 : DataTypeConversion  OutDataTypeStr=uint8  ConvertRealWorld=Stored Integer (SI)
  Direct Lookup Table (n-D) : LookupNDDirect  NumberOfTableDimensions=1  TableIsInput=on
  Direct Lookup Table (n-D)1 : LookupNDDirect  NumberOfTableDimensions=1  TableIsInput=on
  Divide1 : Product  Inputs=*/  OutDataTypeStr=uint16
  Divide2 : Product  Inputs=*/  OutDataTypeStr=uint16
  Relational Operator : RelationalOperator  Operator===  OutDataTypeStr=boolean  RndMeth=Simplest
  Selector{1..4} (4 alike) : Selector  IndexMode=Zero-based  IndexOptions=Index vector (port)  Indices=[1 3]  OutputSizes=1
  Switch : Switch  Criteria=u2 ~= 0
  V_StartGammaValue : Outport  InitialOutput=0  VectorParamsAs1DForOutWhenUnconnected=off
  V_EndGammaValue : Outport  Port=2  InitialOutput=0  VectorParamsAs1DForOutWhenUnconnected=off
  V_NumOfStartSteps : Outport  Port=3  InitialOutput=0  VectorParamsAs1DForOutWhenUnconnected=off
  V_NumOfRampSteps : Outport  Port=4  InitialOutput=0  VectorParamsAs1DForOutWhenUnconnected=off
  wires:
  Add/1 -> Selector3/2
  V_CurrentAnimationStep/1 -> Add2/2
  Add2/1 -> [V_CurrentAnimationStep]
  C_TRamp/1 -> Selector2/1
  [V_CurrentAnimationStep] -> Selector2/2
  C_TStart/1 -> Selector1/1
  [V_CurrentAnimationStep] -> Selector1/2
  C_EndValues/1 -> Selector3/1, Selector4/1
  [V_CurrentAnimationStep] -> Selector4/2
  [V_CurrentAnimationStep] -> Relational Operator/2
  Relational Operator/1 -> [V_IsFirstStep]
  [V_IsFirstStep] -> Switch/2
  Selector3/1 -> Switch/3
  C_StartValues/1 -> Switch/1
  [V_CurrentAnimationStep] -> Add/1
  Constant2/1 -> Add/2
  [C_AnimationPeriod] -> Divide1/2
  Selector2/1 -> Divide1/1
  C_AnimationPeriod/1 -> [C_AnimationPeriod]
  Divide1/1 -> V_NumOfRampSteps/1
  [C_AnimationPeriod] -> Divide2/2
  Selector1/1 -> Divide2/1
  Divide2/1 -> V_NumOfStartSteps/1
  V_IndexOfStartStep/1 -> Relational Operator/1, Add2/1
  C_CieCurvePwmToGammaY/1 -> [C_CieCurvePwmToGammaY]
  Switch/1 -> Data Type Conversion/1
  Data Type Conversion/1 -> Data Type Conversion1/1
  Data Type Conversion1/1 -> Direct Lookup Table (n-D)/1
  [C_CieCurvePwmToGammaY] -> Direct Lookup Table (n-D)/2
  Direct Lookup Table (n-D)/1 -> V_StartGammaValue/1
  [C_CieCurvePwmToGammaY] -> Direct Lookup Table (n-D)1/2
  Data Type Conversion3/1 -> Direct Lookup Table (n-D)1/1
  Data Type Conversion2/1 -> Data Type Conversion3/1
  Selector4/1 -> Data Type Conversion2/1
  Direct Lookup Table (n-D)1/1 -> V_EndGammaValue/1

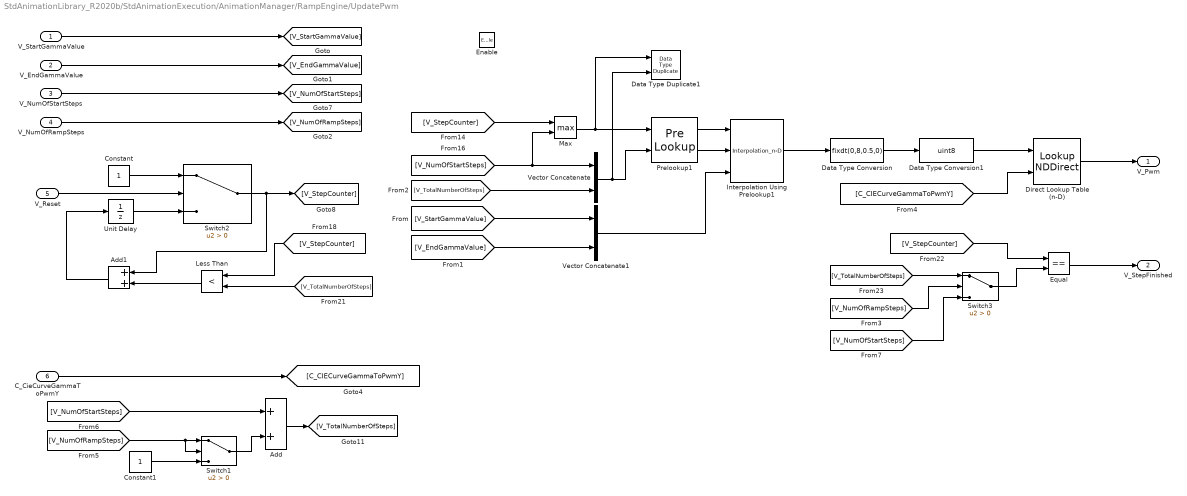
== system StdAnimationLibrary_R2020b/StdAnimationExecution/AnimationManager/RampEngine/UpdatePwm ==
  V_StartGammaValue : Inport
  V_EndGammaValue : Inport  Port=2
  V_NumOfStartSteps : Inport  Port=3
  V_NumOfRampSteps : Inport  Port=4
  V_Reset : Inport  Port=5  OutDataTypeStr=boolean
  C_CieCurveGammaToPwmY : Inport  Port=6
  Enable : EnablePort
  Add : Sum  OutDataTypeStr=Inherit: Inherit via back propagation  SaturateOnIntegerOverflow=on
  Add1 : Sum  OutDataTypeStr=Inherit: Inherit via back propagation  SaturateOnIntegerOverflow=on
  Constant : Constant  OutDataTypeStr=Inherit: Inherit via back propagation
  Constant1 : Constant  OutDataTypeStr=Inherit: Inherit via back propagation
  Data Type Duplicate1 : DataTypeDuplicate
  Data Type Conversion : DataTypeConversion  OutDataTypeStr=fixdt(0,8,0.5,0)  RndMeth=Round
  Data Type Conversion1 : DataTypeConversion  OutDataTypeStr=uint8  ConvertRealWorld=Stored Integer (SI)
  Direct Lookup Table (n-D) : LookupNDDirect  NumberOfTableDimensions=1  TableIsInput=on  RemoveProtectionInput=on
  Equal : RelationalOperator  Operator===  OutDataTypeStr=boolean  RndMeth=Simplest
  Interpolation Using Prelookup1 : Interpolation_n-D  NumberOfTableDimensions=1  TableSource=Input port  ExtrapMethod=Clip  RemoveProtectionIndex=on  ValidIndexMayReachLast=on  InternalRulePriority=Speed
      settings: InputPortMap=u0,u1,p2
  Less Than : RelationalOperator  Operator=<  OutDataTypeStr=boolean  RndMeth=Simplest  InputSameDT=on
  Max : MinMax  Function=max  Inputs=2
  Prelookup1 : PreLookup  BreakpointsDataSource=Input port  BreakpointsData=[10:10:110]  BreakpointObject=P_CIE_GAMMA  IndexSearchMethod=Linear search  BeginIndexSearchUsingPreviousIndexResult=on  UseLastBreakpoint=on  RemoveProtectionInput=on  IndexDataTypeStr=uint16
      settings: InputPortMap=u0,p1
  Switch1 : Switch  Criteria=u2 > Threshold  OutDataTypeStr=Inherit: Inherit via back propagation  SaturateOnIntegerOverflow=on
  Switch2 : Switch  Criteria=u2 > Threshold  OutDataTypeStr=Inherit: Inherit via back propagation
  Switch3 : Switch  Criteria=u2 > Threshold  OutDataTypeStr=Inherit: Inherit via back propagation  SaturateOnIntegerOverflow=on
  Unit Delay : UnitDelay  InitialCondition=1  SampleTime=-1  HasFrameUpgradeWarning=on
  Vector Concatenate : Concatenate
  Vector Concatenate1 : Concatenate
  V_Pwm : Outport  InitialOutput=0  VectorParamsAs1DForOutWhenUnconnected=off
  V_StepFinished : Outport  Port=2  InitialOutput=0  VectorParamsAs1DForOutWhenUnconnected=off
  wires:
  [V_NumOfStartSteps] -> Switch3/3
  Switch3/1 -> Equal/2
  [V_TotalNumberOfSteps] -> Switch3/1
  [V_NumOfRampSteps] -> Switch3/2
  [V_StepCounter] -> Less Than/1
  V_NumOfStartSteps/1 -> [V_NumOfStartSteps]
  [V_NumOfStartSteps] -> Max/2, Vector Concatenate/1
  V_Reset/1 -> Switch2/2
  Unit Delay/1 -> Switch2/3
  Add1/1 -> Unit Delay/1
  V_NumOfRampSteps/1 -> [V_NumOfRampSteps]
  Equal/1 -> V_StepFinished/1
  [V_StepCounter] -> Equal/1
  [V_TotalNumberOfSteps] -> Less Than/2
  Less Than/1 -> Add1/2
  Switch2/1 -> [V_StepCounter], Add1/1
  [V_TotalNumberOfSteps] -> Vector Concatenate/2
  [V_StartGammaValue] -> Vector Concatenate1/1
  [V_EndGammaValue] -> Vector Concatenate1/2
  Direct Lookup Table (n-D)/1 -> V_Pwm/1
  V_StartGammaValue/1 -> [V_StartGammaValue]
  V_EndGammaValue/1 -> [V_EndGammaValue]
  Constant1/1 -> Switch1/3
  Switch1/1 -> Add/2
  Add/1 -> [V_TotalNumberOfSteps]
  C_CieCurveGammaToPwmY/1 -> [C_CIECurveGammaToPwmY]
  Vector Concatenate/1 -> Prelookup1/2, Data Type Duplicate1/2
  [V_NumOfStartSteps] -> Add/1
  [V_NumOfRampSteps] -> Switch1/2, Switch1/1
  Max/1 -> Prelookup1/1, Data Type Duplicate1/1
  [V_StepCounter] -> Max/1
  Vector Concatenate1/1 -> Interpolation Using Prelookup1/3
  Prelookup1/1 -> Interpolation Using Prelookup1/1
  Prelookup1/2 -> Interpolation Using Prelookup1/2
  Interpolation Using Prelookup1/1 -> Data Type Conversion/1
  Data Type Conversion/1 -> Data Type Conversion1/1
  Data Type Conversion1/1 -> Direct Lookup Table (n-D)/1
  [C_CIECurveGammaToPwmY] -> Direct Lookup Table (n-D)/2
  Constant/1 -> Switch2/1
